simulink model "Kalm_5D_2"  (Simulink 8.1)
settings: Solver=FixedStepDiscrete  StartTime=0.0  StopTime=sim_t  FixedStep=0.01  RelTol=1e-3
values from neighbouring files (symbols this model uses):
  A = zeros(34)    [init.m]
  c = [a(2).*b(3)-a(3).*b(2) ... (first row only)    [cross2.m]    (also in ut_weights.m = n + lambda)
  hparamsL = [[arms(3:4), zeros(1,7)]; [m0(3,1:3) xL(1:3) s1P1L']; [m0(4,1:3) xL(4:6) s2P2L']]    [init.m]
  hparamsR = [[arms(1:2), zeros(1,7)]; [m0(1,1:3) xR(1:3) s1P1R']; [m0(2,1:3) xR(4:6) s2P2R']]    [init.m]
  M0 = [zeros(30,1); arm0']    [init.m]
  P0 = diag(repmat(covEps,34,1))    [init.m]
  Q = blkdiag(diag(covQ1), diag(covQ1), diag(covQ1), diag(covQ1), diag(covQ1), diag(covQ1), diag(covQ1), diag(covQ1), diag(covQ1), diag(covQ1), eye(4))    [init.m]
  RR = blkdiag(RL, RR, 1e-6*eye(3),1e-6*eye(3),1e-6*eye(3))    [init.m]
  W = W * diag(WC) * W'    [ut_weights.m]
  WM = zeros(2*n+1,1)    [ut_weights.m]
settings Model: Creator=Lorenzo  LastModifiedBy=Alessandro
settings SolverCC: PositivePriorityOrder=on
settings DataIOCC: SaveOutput=off  SaveTime=off
settings OptimizationCC: OptimizeModelRefInitCode=on  LifeSpan=1
settings DebuggingCC: FcnCallInpInsideContextMsg=EnableAllAsWarning
settings HardwareCC: ProdHWDeviceType=Generic->Unspecified (assume 32-bit Generic)
settings ModelReferenceCC: ModelReferenceMinAlgLoopOccurrences=on
settings RTWCC: SystemTargetFile=idelink_ert.tlc  GenerateMakefile=off  TemplateMakefile=idelink_ert.tmf  Description=IDE Link ERT  ProcessScript=idelink_ert_make_rtw_hook
settings CodeAppCC: IgnoreCustomStorageClasses=off
settings TargetCC: CodeReplacementLibrary=ANSI_C  IsPILTarget=off  CompOptLevelCompliant=off  ConcurrentExecutionCompliant=on  ERTFirstTimeCompliant=on  ERTCustomFileBanners=on  SupportContinuousTime=off  SupportNonInlinedSFcns=off  EnableShiftOperators=on  ModelStepFunctionPrototypeControlCompliant=on
settings CustomProperty: DataType=string

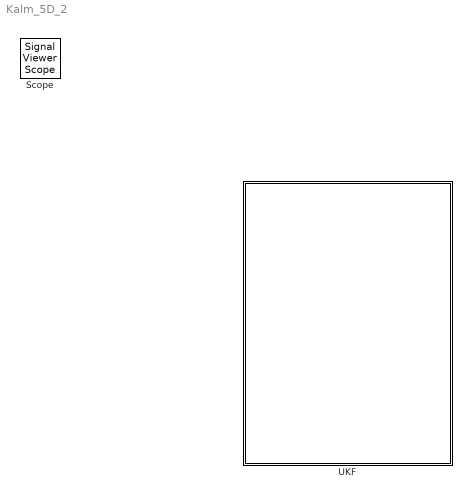
== system Kalm_5D_2 ==
  UKF : Subsystem
  Scope : SignalViewerScope  IOType=viewer  ZoomMode=yonly  RefreshTime=0.035000
      settings: TimeRange=74  YMin=-0.01  YMax=0.12

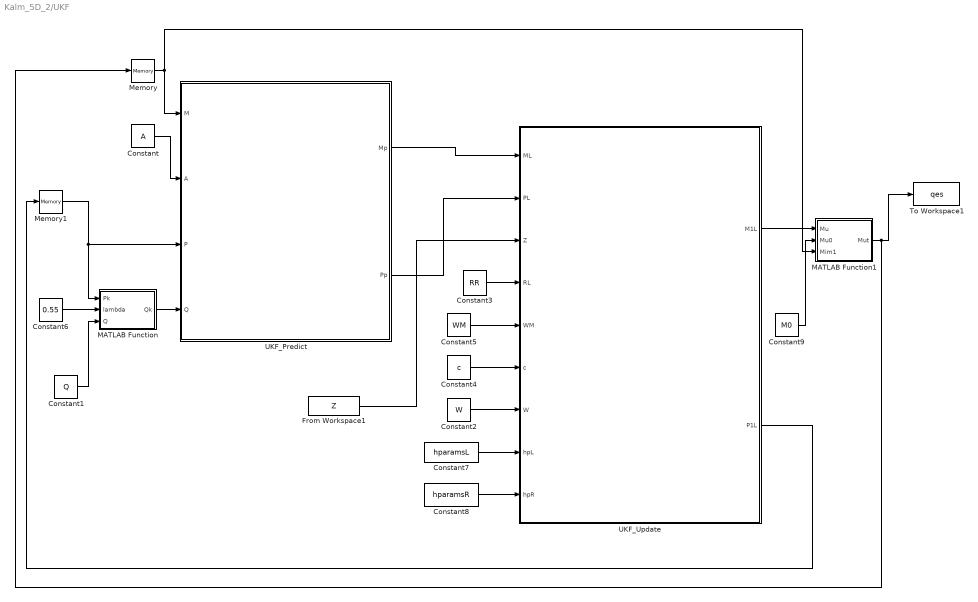
== system Kalm_5D_2/UKF ==
  Constant : Constant  Value=A
  Constant1 : Constant  Value=Q
  Constant2 : Constant  Value=W
  Constant3 : Constant  Value=RR
  Constant4 : Constant  Value=c
  Constant5 : Constant  Value=WM
  Constant6 : Constant  Value=0.55
  Constant7 : Constant  Value=hparamsL
  Constant8 : Constant  Value=hparamsR
  Constant9 : Constant  Value=M0
  From Workspace1 : FromWorkspace  VariableName=Z  SampleTime=0.01  Interpolate=off  OutputAfterFinalValue=Holding final value
  MATLAB Function : MATLAB Function  TreatAsAtomicUnit=on
  MATLAB Function1 : MATLAB Function  TreatAsAtomicUnit=on
  Memory : Memory  X0=M0
  Memory1 : Memory  X0=P0
  To Workspace1 : ToWorkspace  VariableName=qes  SampleTime=-1  SaveFormat=Structure
  UKF_Predict : Subsystem
  UKF_Update : Subsystem
  wires:
  Memory/1 -> MATLAB Function1/3(Mim1), UKF_Predict/1(M)
  Constant5/1 -> UKF_Update/5(WM)
  Constant2/1 -> UKF_Update/7(W)
  UKF_Update/2(P1L) -> Memory1/1
  Constant4/1 -> UKF_Update/6(c)
  Constant8/1 -> UKF_Update/9(hpR)
  Constant/1 -> UKF_Predict/2(A)
  Memory1/1 -> MATLAB Function/1(Pk), UKF_Predict/3(P)
  From Workspace1/1 -> UKF_Update/3(Z)
  UKF_Predict/2(Pp) -> UKF_Update/2(PL)
  Constant7/1 -> UKF_Update/8(hpL)
  Constant3/1 -> UKF_Update/4(RL)
  MATLAB Function/1(Qk) -> UKF_Predict/4(Q)
  UKF_Predict/1(Mp) -> UKF_Update/1(ML)
  Constant1/1 -> MATLAB Function/3(Q)
  Constant6/1 -> MATLAB Function/2(lambda)
  UKF_Update/1(M1L) -> MATLAB Function1/1(Mu)
  MATLAB Function1/1(Mut) -> Memory/1, To Workspace1/1
  Constant9/1 -> MATLAB Function1/2(Mu0)

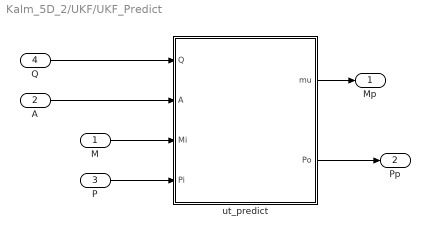
== system Kalm_5D_2/UKF/UKF_Predict ==
  M : Inport
  A : Inport  Port=2
  P : Inport  Port=3
  Q : Inport  Port=4
  ut_predict : MATLAB Function  TreatAsAtomicUnit=on
  Mp : Outport
  Pp : Outport  Port=2
  wires:
  ut_predict/1(mu) -> Mp/1
  ut_predict/2(Po) -> Pp/1
  A/1 -> ut_predict/2(A)
  Q/1 -> ut_predict/1(Q)
  M/1 -> ut_predict/3(Mi)
  P/1 -> ut_predict/4(Pi)

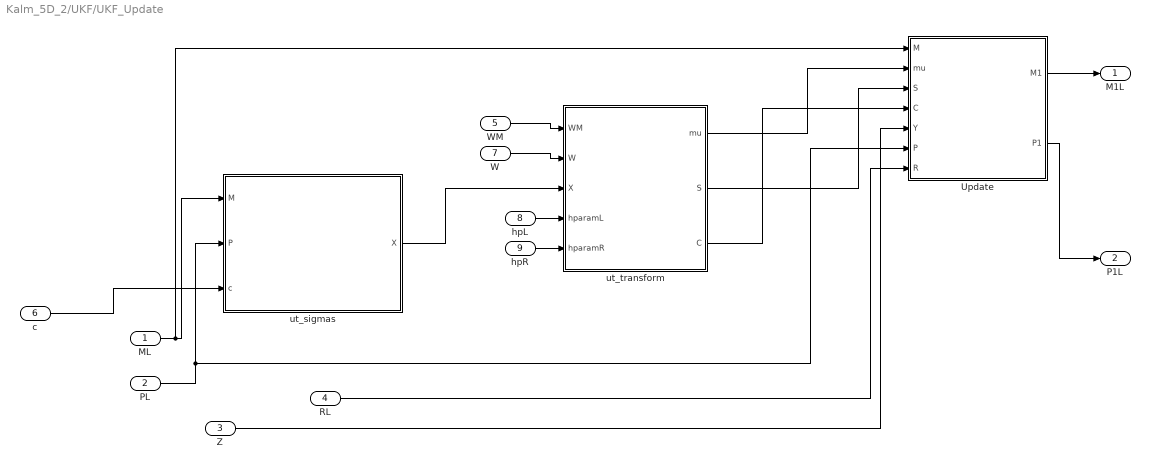
== system Kalm_5D_2/UKF/UKF_Update ==
  ML : Inport
  PL : Inport  Port=2
  Z : Inport  Port=3
  RL : Inport  Port=4
  WM : Inport  Port=5
  c : Inport  Port=6
  W : Inport  Port=7
  hpL : Inport  Port=8
  hpR : Inport  Port=9
  Update : MATLAB Function  TreatAsAtomicUnit=on
  ut_sigmas : MATLAB Function  TreatAsAtomicUnit=on
  ut_transform : MATLAB Function  TreatAsAtomicUnit=on
  M1L : Outport
  P1L : Outport  Port=2
  wires:
  ut_sigmas/1(X) -> ut_transform/3(X)
  PL/1 -> ut_sigmas/2(P), Update/6(P)
  ML/1 -> ut_sigmas/1(M), Update/1(M)
  ut_transform/1(mu) -> Update/2(mu)
  ut_transform/2(S) -> Update/3(S)
  ut_transform/3(C) -> Update/4(C)
  Z/1 -> Update/5(Y)
  Update/2(P1) -> P1L/1
  RL/1 -> Update/7(R)
  Update/1(M1) -> M1L/1
  WM/1 -> ut_transform/1(WM)
  W/1 -> ut_transform/2(W)
  c/1 -> ut_sigmas/3(c)
  hpL/1 -> ut_transform/4(hparamL)
  hpR/1 -> ut_transform/5(hparamR)

== matlab function UKF/UKF_Predict/ut_predict ==
  data: Q input double; mu output double; A input double; Po output double; Mi input double; Pi input double
function [mu,Po] = ut_predict(Q,A,Mi,Pi)
%#codegen
      
  %
  % Calculate sigma points
  %
  
%   w = {WM,WC,c};
  
  %
  % Propagate through the function
  %
  mu = A*Mi;
  Po = A*Pi*A'+Q;
end

== matlab function UKF/UKF_Update/ut_transform ==
  data: mu output double; WM input double; W input double; S output double; X input double; C output double; hparamL input double; hparamR input double
function [mu,S,C] = ut_transform_h(WM,W,X, hparamL, hparamR)
%#codegen
      
  %
  % Calculate sigma points
  %
  
%   w = {WM,WC,c};
  
  %
  % Propagate through the function
  %
  
  Y = zeros(45,69);
  for i=1:size(X,2)
      Y(1:18,i) = hn_sim5DL(X(1:15,i), X(31:32,i), hparamL);
      Y(19:36,i) = hn_sim5DR(X(16:30,i), X(33:34,i), hparamR);
      Y(37:45,i) = paramH(X(:,i));
  end
  
  
  mu = Y*WM;
  S  = Y*W*Y';
  C  = X*W*Y';
  
  
  end

== matlab function UKF/MATLAB Function ==
  data: Pk input double; Qk output double; lambda input double; Q input double
function Qk = Q_gen(Pk, lambda, Q)
%#codegen

th = 1e-15;
Qk = Q;
Qp = (1/lambda - 1)*Pk(31:34,31:34);
if det(Qp) < th
    Qk(31:34,31:34) = 1e-15*eye(4);
else
    Qk(31:34,31:34) = Qp;
end

end

== matlab function UKF/MATLAB Function1 ==
  data: Mu input double; Mut output double; Mu0 input double; Mim1 input double
function Mut = M_thr(Mu, Mu0, Mim1)
%#codegen

th = 0.1;
Mut = Mu;
Mut(1:3:30) = atan2(sin(Mut(1:3:30)),cos(Mut(1:3:30)));
if norm(Mut(31:34) - Mu0(31:34)) > th
    Mut(31:34) = Mim1(31:34);
end


end

== matlab function UKF/UKF_Update/ut_sigmas ==
  data: M input double; X output double; P input double; c input double
function X = ut_sigmas(M,P,c)

%#codegen
A = chol(P)';
X = [zeros(size(M)) A -A];
X = sqrt(c)*X + repmat(M,1,size(X,2));

== matlab function UKF/UKF_Update/Update ==
  data: M input double; M1 output double; mu input double; S input double; C input double; Y input double; P input double; P1 output double; R input double
function [M1, P1] = update(M,mu, S, C, Y, P, R)
%#codegen
S = S+R;
K = C/S;
M1 = M+K*(Y-mu);
P1 = P-K*S*K';
